simulink model "my_pv_system_3_ss_calculation"  (Simulink 8.4)
settings: Solver=ode3  StartTime=0.0  StopTime=inf  FixedStep=5e-05  RelTol=1e-3
libraries: opal_lib x5, powerlib_meascontrol x2, powerlib x1
Description:
  | Model of a simple control system for use iin training.
settings Model: Creator=Paul Baracos  LastModifiedBy=jiang  BufferReuse=off
settings DataIOCC: SaveOutput=off  SaveTime=off  SignalLoggingName=sigsOut
settings OptimizationCC: BlockReduction=off  BooleanDataType=off  OptimizeBlockIOStorage=off  BufferReuse=off  GlobalBufferReuse=off  ExpressionFolding=off  ExpressionDepthLimit=128  LocalBlockOutputs=off  InitFltsAndDblsToZero=on
settings DebuggingCC: SaveWithParameterizedLinksMsg=none  SignalResolutionControl=TryResolveAllWithWarning  SolverPrmCheckMsg=none  MultiTaskDSMMsg=warning  MultiTaskCondExecSysMsg=none  StateNameClashWarn=none
settings HardwareCC: TargetHWDeviceType=32-bit Generic  TargetUnknown=on  ProdEqTarget=off
settings RTWCC: GenCodeOnly=on  IncludeERTFirstTime=on
settings GRTTargetCC: TargetFcnLib=ansi_tfl_tmw.mat
settings ConfigurationSet: Description=SimMechanics 2G

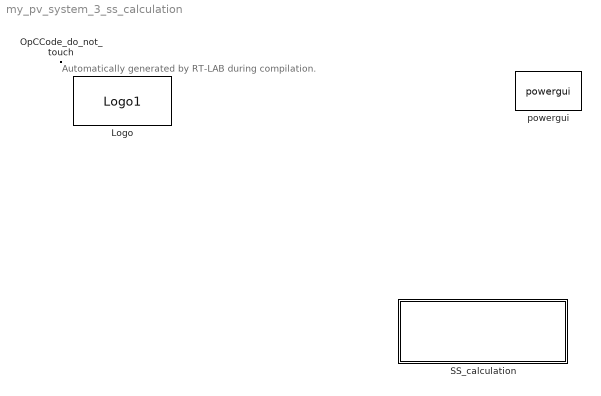
== system my_pv_system_3_ss_calculation ==
  note: Automatically generated by RT-LAB during compilation.
  Logo : opal_lib/Logo1  vide=[]
  OpCCode_do_not_touch : opal_lib/Communication/OpCCode  SystemSampleTime=-1
  SS_calculation : Subsystem
  powergui : powerlib/powergui  SimulationMode=Discrete  SolverType=Tustin/Backward Euler (TBE)  SampleTime=5e-05  frequency=60  SPID=off  DisableSnubberDevices=off  DisableRonSwitches=off  DisableVfSwitches=off  SwTol=0  DisplayEquations=off  Interpol=off  methode=off  Ts=100  frequencyindice=50  Pbase=100e6  ErrMax=1e-4  Iterations=50  UnitsV=kV  UnitsW=MW  FunctionMessages=off  echomessages=off  HookPort=off  EnableUseOfTLC=off  x0status=blocks  RestoreLinks=warning  ResistiveCurrentMeasurement=off  Frange=[0:2:500]  Ylog=off  Xlog=on  ShowGrid=off  save=off  variable=ZData  structure=0  ZoomFFT=off  StartTime=0.0  cycles=1  DisplayStyle=1  fundamental=60  FreqAxis=off  MaxFrequency=1000  frequencyindicesteady=1  RmsSteady=1  display=off

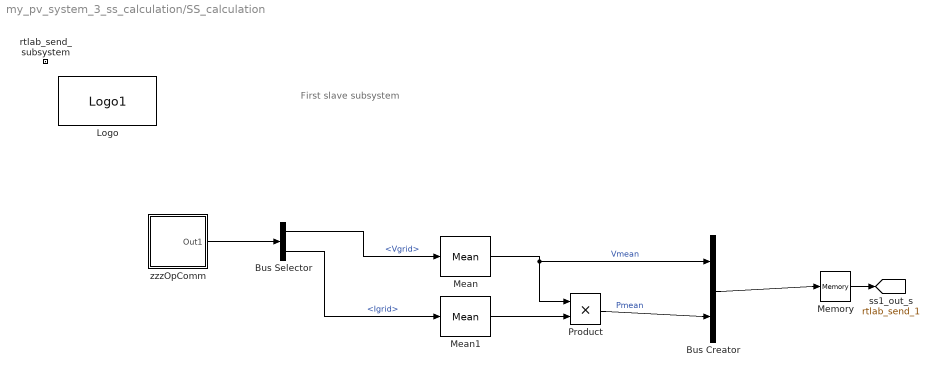
== system my_pv_system_3_ss_calculation/SS_calculation ==
  note: First slave subsystem
  Bus Creator : BusCreator  Inputs=2
  Bus Selector : BusSelector  OutputSignals=Vgrid,Igrid
  Logo : opal_lib/Logo1  vide=[]
  Mean : powerlib_meascontrol/Measurements/Mean  Freq=50  Vinit=0  Ts=50e-6
  Mean1 : powerlib_meascontrol/Measurements/Mean  Freq=50  Vinit=0  Ts=50e-6
  Memory : Memory  InheritSampleTime=on
  Product : Product
  rtlab_send_subsystem : Subsystem  Priority=-100
      mask Display: text(0,0,'');
  zzzOpComm : Subsystem
      mask init:
      | opmaskdisplay('maskdisplay_block',gcb,'disp(''OpComm'')');
      mask Display:
      | patch([0 0.5 0.7 0],[1 1 0 0],[0.7 0.75 0.9]);
      | patch([1 0.53 0.73 1],[1 1 0 0],[1 0.8 0.7]);
      | plot([0 0 1 1 0],[0 1 1 0 0]);
      | disp('OpComm')
  tag scope: rtlab_send_1=global
  wires:
  Memory/1 -> [rtlab_send_1]
  Mean/1 -> Product/1, Bus Creator/1  "Vmean"
  Mean1/1 -> Product/2
  Product/1 -> Bus Creator/2  "Pmean"
  Bus Creator/1 -> Memory/1
  zzzOpComm/1(Out1) -> Bus Selector/1
  Bus Selector/1 -> Mean/1  "<Vgrid>"
  Bus Selector/2 -> Mean1/1  "<Igrid>"

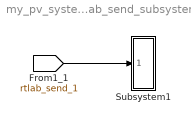
== system my_pv_system_3_ss_calculation/SS_calculation/rtlab_send_subsystem ==
  Subsystem1 : Subsystem
  wires:
  [rtlab_send_1] -> Subsystem1/1(In1)

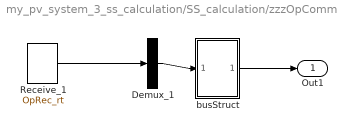
== system my_pv_system_3_ss_calculation/SS_calculation/zzzOpComm ==
  Demux_1 : Demux  Outputs=[5]
  Receive_1 : opal_lib/Communication/OpRec_rt  src=1  Data_width=5  st=5e-05
  busStruct : Subsystem
  Out1 : Outport
  wires:
  Demux_1/1 -> busStruct/1(In1)
  busStruct/1(Out1) -> Out1/1
  Receive_1/1 -> Demux_1/1

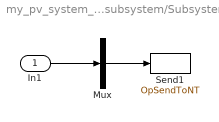
== system my_pv_system_3_ss_calculation/SS_calculation/rtlab_send_subsystem/Subsystem1 ==
  In1 : Inport
  Mux : Mux  Inputs=1
  Send1 : opal_lib/Communication/OpSendToNT  Acqu_group=1
  wires:
  Mux/1 -> Send1/1
  In1/1 -> Mux/1

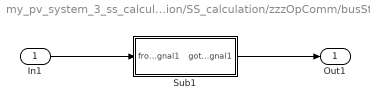
== system my_pv_system_3_ss_calculation/SS_calculation/zzzOpComm/busStruct ==
  In1 : Inport
  Sub1 : Subsystem
  Out1 : Outport
  wires:
  Sub1/1(goto_signal1) -> Out1/1
  In1/1 -> Sub1/1(from_signal1)

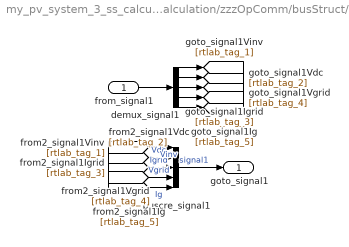
== system my_pv_system_3_ss_calculation/SS_calculation/zzzOpComm/busStruct/Sub1 ==
  from_signal1 : Inport
  buscre_signal1 : BusCreator  Inputs=5
  demux_signal1 : Demux  Outputs="[1  1  1  1  1]"
  goto_signal1 : Outport
  wires:
  buscre_signal1/1 -> goto_signal1/1  "signal1"
  [rtlab_tag_5] -> buscre_signal1/5  "Ig"
  [rtlab_tag_4] -> buscre_signal1/4  "Vgrid"
  [rtlab_tag_3] -> buscre_signal1/3  "Igrid"
  [rtlab_tag_2] -> buscre_signal1/2  "Vdc"
  [rtlab_tag_1] -> buscre_signal1/1  "Vinv"
  demux_signal1/5 -> [rtlab_tag_5]
  demux_signal1/4 -> [rtlab_tag_4]
  demux_signal1/3 -> [rtlab_tag_3]
  demux_signal1/2 -> [rtlab_tag_2]
  demux_signal1/1 -> [rtlab_tag_1]
  from_signal1/1 -> demux_signal1/1
